simulink model "test_scenario"  (R2026a)
settings: Solver=FixedStepDiscrete  StopTime=inf  FixedStep=1/250
values from neighbouring files (symbols this model uses):
  amplitude_1 = 20e-6    (= 2e-05)    [STUBSCRIPT.m]    (also in main.m; main_calibrazione.m; profilazione.m; setup.m)
  amplitude_2 = 30e-6    (= 3e-05)    [STUBSCRIPT.m]    (also in main.m; main_calibrazione.m; profilazione.m; setup.m)
  amplitude_3 = 40e-6    (= 4e-05)    [STUBSCRIPT.m]    (also in main.m; main_calibrazione.m; profilazione.m; setup.m)
  amplitude_4 = 50e-6    (= 5e-05)    [STUBSCRIPT.m]    (also in main.m; main_calibrazione.m; profilazione.m; setup.m)
  unicorn_buff_size = 25    [STUBSCRIPT.m]    (also in main.m; main_calibrazione.m; profilazione.m; setup.m)
  unicorn_f = 250    [STUBSCRIPT.m]    (also in main.m; main_calibrazione.m; profilazione.m; setup.m)
undefined symbols (not defined in the file or in its folder): fdesignblkfcn, gcbh, UN
libraries: simulink x10, dspfdesign x8, dsparch4 x2, UnicornLib x1
settings Model: Creator=Utente  LastModifiedBy=Flexo Rodriguez

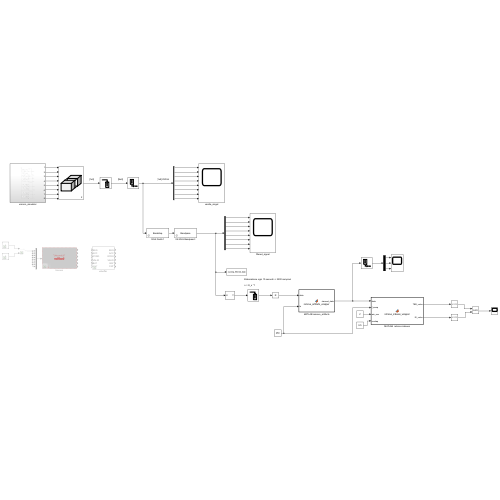
[thumbnail: Simulink's stored preview of the top-level diagram]
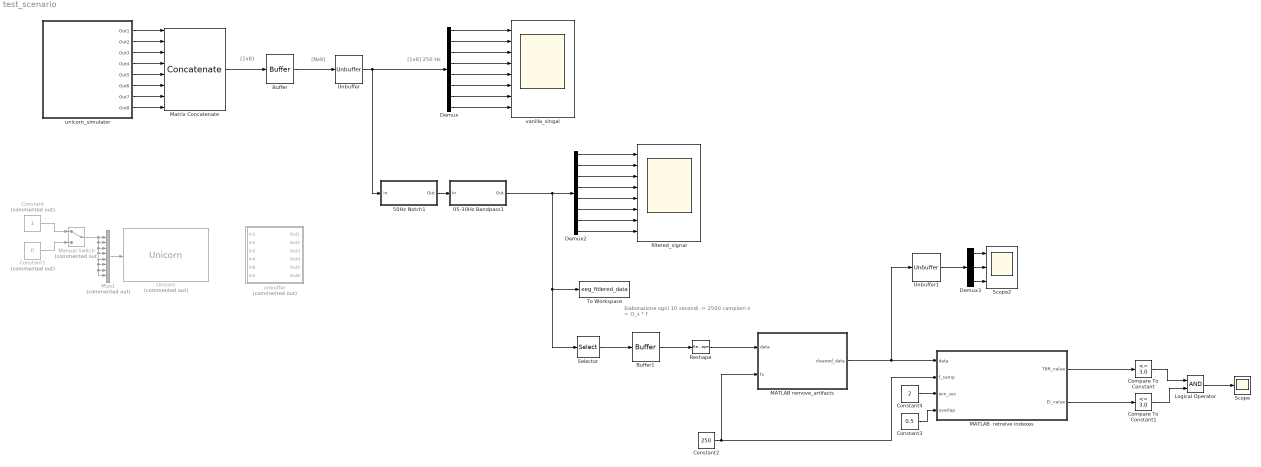
== system test_scenario ==
  note: Elaborazione ogni 10 secondi -> 2500 campioni
      |
      | n = O_s * f
  note: [1x8] 250 Hz
  note: [1x8]
  note: [Nx8]
  05-30Hz Bandpass1 : Subsystem  DialogController=fdesignblkfcn  InitFcn=fdesignblkfcn(gcbh, {'InitFcn'});  mask(Bandpass Filter){}
      mask help: Design a bandpass filter
      settings: CopyFcn=fdesignblkfcn(gcbh, {'CopyFcn'});
      mask Help: helpview(mapfilelocation('dsp'), 'dspbandpassfilter');
      mask Display: disp('Bandpass');
  50Hz Notch1 : Subsystem  DialogController=fdesignblkfcn  InitFcn=fdesignblkfcn(gcbh, {'InitFcn'});  mask(Bandstop Filter){}
      mask help: Design a bandstop filter
      settings: CopyFcn=fdesignblkfcn(gcbh, {'CopyFcn'});
      mask Help: helpview(mapfilelocation('dsp'), 'dspbandstopfilter');
      mask Display: disp('Bandstop');
  Buffer : Buffer  N=unicorn_buff_size  OutputFrames=off
  Buffer1 : Buffer  N=2500  OutputFrames=off
  Compare To Constant : simulink/Logic and Bit Operations/Compare To Constant  relop=<=  const=3.0  OutDataTypeStr=boolean
  Compare To Constant1 : simulink/Logic and Bit Operations/Compare To Constant  relop=<=  const=3.0  OutDataTypeStr=boolean
  Constant : Constant  Commented=on  OutDataTypeStr=boolean
  Constant1 : Constant  Commented=on  Value=0  OutDataTypeStr=boolean
  Constant2 : Constant  Value=250
  Constant3 : Constant  Value=0.5
  Constant4 : Constant  Value=2
  Demux : Demux  Outputs=8
  Demux2 : Demux  Outputs=8
  Demux3 : Demux  Outputs=3
  Logical Operator : Logic  AllPortsSameDT=off  OutDataTypeStr=boolean
  MATLAB  retreive indexes : MATLAB Function  TreatAsAtomicUnit=on
  MATLAB remove_artifacts : MATLAB Function  TreatAsAtomicUnit=on
  Manual Switch : ManualSwitch  Commented=on
  Matrix Concatenate : Concatenate  NumInputs=8  Mode=Multidimensional array  ConcatenateDimension=2
  Mux1 : Mux  Commented=on  Inputs=8
  Reshape : Reshape  OutputDimensionality=Customize  OutputDimensions=[2500,3]
  Scope : Scope
      settings: ActiveDisplayYMinimum=-1.7587335074953709  ActiveDisplayYMaximum=3.3735192626757464  DataLoggingVariableName=ScopeData2
  Scope2 : Scope  NumInputPorts=3
      settings: ActiveDisplayYMinimum=-2.8982593996217672  ActiveDisplayYMaximum=3.2740071294461224  DataLoggingVariableName=ScopeData4
  Selector : Selector  InputPortWidth=8  IndexOptions=Index vector (dialog)  Indices=[1 3 5]  OutputSizes=1
  To Workspace : ToWorkspace  VariableName=eeg_fitlered_data  SampleTime=-1
      settings: Save2DSignal=2-D array (concatenate along first dimension)
  Unbuffer : Unbuffer
  Unbuffer1 : Unbuffer
  Unicorn : UnicornLib/Unicorn  Commented=on  serial=UN-2023.04.40  old_serial=UN-2023.04.40  frame_length=1  input_source=Electrode
      settings: SourceProductName=Unicorn
  filtered_signal : Scope  NumInputPorts=8
      settings: ActiveDisplayYMinimum=-0.11132567955130231  ActiveDisplayYMaximum=0.12003241029464064  DataLoggingVariableName=ScopeData3
  "unbuffer " : Subsystem  Commented=on
      mask Display:
      | port_label('input',1,'EEG')
      | port_label('input',2,'ACC')
      | port_label('input',3,'GYRO')
      | port_label('input',4,'VALID')
      | port_label('input',5,'BAT')
      | port_label('input',6,'CNT')
      | port_label('output',1,'EEG')
      | port_label('output',2,'ACC')
      | port_label('output',3,'GYRO')
      | port_label('output',4,'VALID')
      | port_label('output',5,'BAT')
      | port_label('output',6,'CNT')
  unicorn_simulator : Subsystem
  vanilla_singal : Scope  NumInputPorts=8
      settings: ActiveDisplayString=4  ActiveDisplayYMinimum=-0.17938110629942738  ActiveDisplayYMaximum=0.15369010614959708
  wires:
  Constant/1 -> Manual Switch/1
  Mux1/1 -> Unicorn/1
  Manual Switch/1 -> Mux1/8, Mux1/7, Mux1/6, Mux1/5, Mux1/4, Mux1/3, Mux1/2, Mux1/1
  Constant1/1 -> Manual Switch/2
  unicorn_simulator/1(Out1) -> Matrix Concatenate/1
  unicorn_simulator/2(Out2) -> Matrix Concatenate/2
  unicorn_simulator/3(Out3) -> Matrix Concatenate/3
  unicorn_simulator/4(Out4) -> Matrix Concatenate/4
  unicorn_simulator/5(Out5) -> Matrix Concatenate/5
  unicorn_simulator/6(Out6) -> Matrix Concatenate/6
  unicorn_simulator/7(Out7) -> Matrix Concatenate/7
  unicorn_simulator/8(Out8) -> Matrix Concatenate/8
  Matrix Concatenate/1 -> Buffer/1
  Buffer/1 -> Unbuffer/1
  Unbuffer/1 -> Demux/1, 50Hz Notch1/1(In)
  Demux/1 -> vanilla_singal/1
  Demux/3 -> vanilla_singal/3
  Demux/2 -> vanilla_singal/2
  Demux/4 -> vanilla_singal/4
  Demux/5 -> vanilla_singal/5
  Demux/6 -> vanilla_singal/6
  Demux/7 -> vanilla_singal/7
  Demux/8 -> vanilla_singal/8
  50Hz Notch1/1(Out) -> 05-30Hz Bandpass1/1(In)
  05-30Hz Bandpass1/1(Out) -> Selector/1, To Workspace/1, Demux2/1
  Demux2/8 -> filtered_signal/8
  Demux2/3 -> filtered_signal/3
  Demux2/1 -> filtered_signal/1
  Demux2/7 -> filtered_signal/7
  Demux2/2 -> filtered_signal/2
  Demux2/4 -> filtered_signal/4
  Demux2/6 -> filtered_signal/6
  Demux2/5 -> filtered_signal/5
  Selector/1 -> Buffer1/1
  Constant2/1 -> MATLAB  retreive indexes/2(f_samp), MATLAB remove_artifacts/2(fs)
  MATLAB remove_artifacts/1(cleaned_data) -> Unbuffer1/1, MATLAB  retreive indexes/1(data)
  Constant4/1 -> MATLAB  retreive indexes/3(win_sec)
  Constant3/1 -> MATLAB  retreive indexes/4(overlap)
  Compare To Constant/1 -> Logical Operator/1
  Compare To Constant1/1 -> Logical Operator/2
  MATLAB  retreive indexes/1(TBR_value) -> Compare To Constant/1
  MATLAB  retreive indexes/2(EI_value) -> Compare To Constant1/1
  Logical Operator/1 -> Scope/1
  Buffer1/1 -> Reshape/1
  Reshape/1 -> MATLAB remove_artifacts/1(data)
  Demux3/1 -> Scope2/1
  Demux3/2 -> Scope2/2
  Demux3/3 -> Scope2/3
  Unbuffer1/1 -> Demux3/1

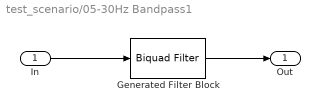
== system test_scenario/05-30Hz Bandpass1 ==
  In : Inport
  Generated Filter Block : dsparch4/Biquad Filter  Tag=BlockMethodSubSystem  FilterSource=Dialog parameters  CoeffSource=Specify via dialog  FilterObject=Hm_biquad  IIRFiltStruct=Direct form II  BiQuadCoeffs=[0.4322526152450743 0 -0.4322526152450743 1 -1.0011806751735479 0.3599418394747359;0.089147308745349971 0 -0.089147308745349971 1 -0.90316691443797437 0.21573805671244461;0.0088211325061849071 0 -0.0088211325061849071 1 -1.9935355151831708 0.99369356215971294;0.012337659349727709 0 -0.012337659349727709 1 -1.9822422643876501 0.98240374527709184;2 0 -2 1 -1.9751756853515128 0.97534142261558909;2 0 -2 1 -1.2458737431168365 0.70689135033598349]  ScaleValues=[0.35278894395693888;1;1;1;1;1;133.18750137787509]  IC=0  ICnum=0  ICden=0  a0Flag=Warning  optimizeScaleValues=on  ScaleValueMode=Specify via input port (g)  roundingMode=Floor  overflowMode=off  scaleValueFracLength=14  denProdOutputFracLength=30  denAccumFracLength=30  secondMemoryFracLength=15
  Out : Outport
  wires:
  In/1 -> Generated Filter Block/1
  Generated Filter Block/1 -> Out/1

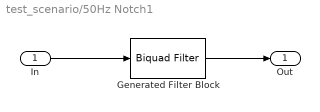
== system test_scenario/50Hz Notch1 ==
  In : Inport
  Generated Filter Block : dsparch4/Biquad Filter  Tag=BlockMethodSubSystem  FilterSource=Dialog parameters  CoeffSource=Specify via dialog  FilterObject=Hm_biquad  IIRFiltStruct=Direct form II  BiQuadCoeffs=[2 -1.2376311593598059 1.9999999999999996 1 -0.58917542534408363 0.90420359373902093]  ScaleValues=[0.091083863875771748;5.226511899890804]  IC=0  ICnum=0  ICden=0  a0Flag=Warning  optimizeScaleValues=on  ScaleValueMode=Specify via input port (g)  roundingMode=Floor  overflowMode=off  scaleValueFracLength=14  denProdOutputFracLength=30  denAccumFracLength=30  secondMemoryFracLength=15
  Out : Outport
  wires:
  Generated Filter Block/1 -> Out/1
  In/1 -> Generated Filter Block/1

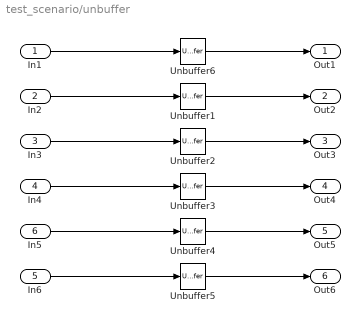
== system test_scenario/unbuffer  ==
  In1 : Inport
  In2 : Inport  Port=2
  In3 : Inport  Port=3
  In4 : Inport  Port=4
  In6 : Inport  Port=5
  In5 : Inport  Port=6
  Unbuffer{1..6} (6 alike) : Unbuffer
  Out1 : Outport
  Out2 : Outport  Port=2
  Out3 : Outport  Port=3
  Out4 : Outport  Port=4
  Out5 : Outport  Port=5
  Out6 : Outport  Port=6
  wires:
  In1/1 -> Unbuffer6/1
  In6/1 -> Unbuffer5/1
  In2/1 -> Unbuffer1/1
  In3/1 -> Unbuffer2/1
  In4/1 -> Unbuffer3/1
  In5/1 -> Unbuffer4/1
  Unbuffer4/1 -> Out5/1
  Unbuffer5/1 -> Out6/1
  Unbuffer3/1 -> Out4/1
  Unbuffer2/1 -> Out3/1
  Unbuffer1/1 -> Out2/1
  Unbuffer6/1 -> Out1/1

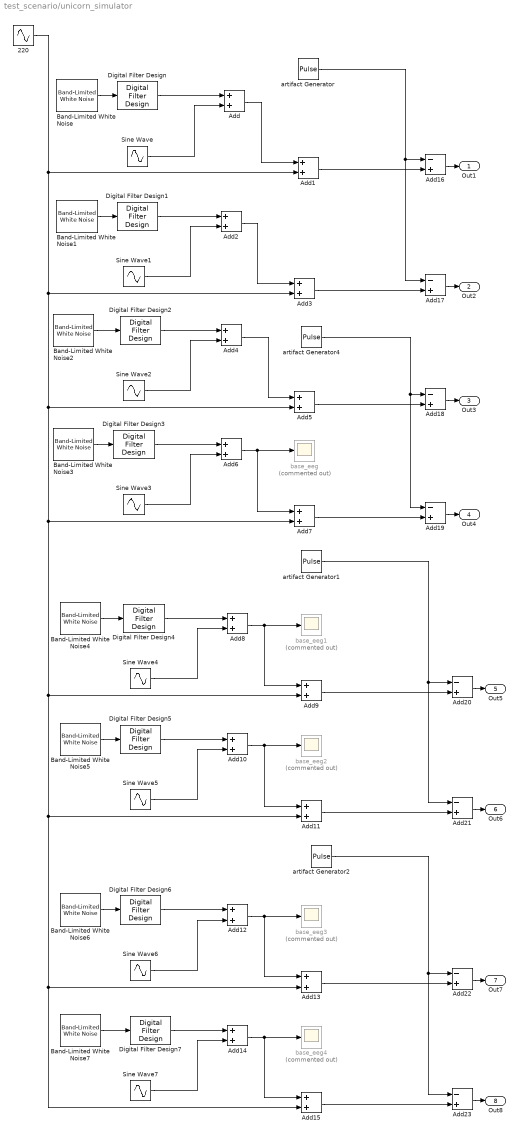
== system test_scenario/unicorn_simulator ==
  220 : Sin  SineType=Sample based  Amplitude=12e-6  Frequency=314.15  SampleTime=1/unicorn_f
  Add{,1..15} (16 alike) : Sum
  Add{16..23} (8 alike) : Sum  Inputs=-+
  Band-Limited White Noise : simulink/Sources/Band-Limited White Noise  Cov=[0.00001]  Ts=1/unicorn_f  seed=[23344]
  Band-Limited White Noise1 : simulink/Sources/Band-Limited White Noise  Cov=[0.00001]  Ts=1/unicorn_f  seed=[23344]
  Band-Limited White Noise2 : simulink/Sources/Band-Limited White Noise  Cov=[0.00001]  Ts=1/unicorn_f  seed=[23343]
  Band-Limited White Noise3 : simulink/Sources/Band-Limited White Noise  Cov=[0.00001]  Ts=1/unicorn_f  seed=[23343]
  Band-Limited White Noise4 : simulink/Sources/Band-Limited White Noise  Cov=[0.00001]  Ts=1/unicorn_f  seed=[23342]
  Band-Limited White Noise5 : simulink/Sources/Band-Limited White Noise  Cov=[0.00001]  Ts=1/unicorn_f  seed=[23342]
  Band-Limited White Noise6 : simulink/Sources/Band-Limited White Noise  Cov=[0.00001]  Ts=1/unicorn_f  seed=[23341]
  Band-Limited White Noise7 : simulink/Sources/Band-Limited White Noise  Cov=[0.00001]  Ts=1/unicorn_f  seed=[23341]
  Digital Filter Design{,1..7} (8 alike) : dspfdesign/Digital Filter Design  mwdsp_browser_bugfix_var=off
  Sine Wave : Sin  SineType=Sample based  Amplitude=amplitude_1  Frequency=62.83  SampleTime=1/unicorn_f
  Sine Wave1 : Sin  SineType=Sample based  Amplitude=amplitude_1  Frequency=62.83  SampleTime=1/unicorn_f
  Sine Wave2 : Sin  SineType=Sample based  Amplitude=amplitude_2  Frequency=62.83  SampleTime=1/unicorn_f
  Sine Wave3 : Sin  Amplitude=amplitude_2  Frequency=62.83  SampleTime=1/unicorn_f
  Sine Wave4 : Sin  SineType=Sample based  Amplitude=amplitude_3  Frequency=62.83  SampleTime=1/unicorn_f
  Sine Wave5 : Sin  SineType=Sample based  Amplitude=amplitude_3  Frequency=62.83  SampleTime=1/unicorn_f
  Sine Wave6 : Sin  SineType=Sample based  Amplitude=amplitude_4  Frequency=62.83  SampleTime=1/unicorn_f
  Sine Wave7 : Sin  SineType=Sample based  Amplitude=amplitude_4  Frequency=62.83  SampleTime=1/unicorn_f
  artifact Generator : DiscretePulseGenerator  Amplitude=1000*amplitude_1  Period=25000*(1/unicorn_f)  PulseWidth=30  SampleTime=1/unicorn_f
  artifact Generator1 : DiscretePulseGenerator  Amplitude=1000*amplitude_3  Period=25000*(1/unicorn_f)  PulseWidth=30  SampleTime=1/unicorn_f
  artifact Generator2 : DiscretePulseGenerator  Amplitude=1000*amplitude_4  Period=25000*(1/unicorn_f)  PulseWidth=30  SampleTime=1/unicorn_f
  artifact Generator4 : DiscretePulseGenerator  Amplitude=1000*amplitude_2  Period=25000*(1/unicorn_f)  PulseWidth=30  SampleTime=1/unicorn_f
  base_eeg{,1..4} (5 alike) : Scope  Commented=on
      base_eeg settings: ActiveDisplayYMinimum=-0.035555269827580581  ActiveDisplayYMaximum=0.026072132085607332
      base_eeg1 settings: ActiveDisplayYMinimum=-0.035555269827580581  ActiveDisplayYMaximum=0.026072132085607332  DataLoggingVariableName=ScopeData5
      base_eeg2 settings: ActiveDisplayYMinimum=-0.035555269827580581  ActiveDisplayYMaximum=0.026072132085607332  DataLoggingVariableName=ScopeData7
      base_eeg3 settings: ActiveDisplayYMinimum=-0.035555269827580581  ActiveDisplayYMaximum=0.026072132085607332  DataLoggingVariableName=ScopeData9
      base_eeg4 settings: ActiveDisplayYMinimum=-0.035555269827580581  ActiveDisplayYMaximum=0.026072132085607332  DataLoggingVariableName=ScopeData11
  Out1 : Outport
  Out2 : Outport  Port=2
  Out3 : Outport  Port=3
  Out4 : Outport  Port=4
  Out5 : Outport  Port=5
  Out6 : Outport  Port=6
  Out7 : Outport  Port=7
  Out8 : Outport  Port=8
  wires:
  Add1/1 -> Add16/2
  Digital Filter Design2/1 -> Add4/1
  Band-Limited White Noise7/1 -> Digital Filter Design7/1
  Sine Wave/1 -> Add/2
  Digital Filter Design4/1 -> Add8/1
  Add/1 -> Add1/1
  Digital Filter Design1/1 -> Add2/1
  220/1 -> Add15/2, Add13/2, Add11/2, Add9/2, Add7/2, Add5/2, Add3/2, Add1/2
  Digital Filter Design6/1 -> Add12/1
  Band-Limited White Noise6/1 -> Digital Filter Design6/1
  Add5/1 -> Add18/2
  Add18/1 -> Out3/1
  Add20/1 -> Out5/1
  artifact Generator4/1 -> Add19/1, Add18/1
  Sine Wave1/1 -> Add2/2
  Sine Wave3/1 -> Add6/2
  Add9/1 -> Add20/2
  Add16/1 -> Out1/1
  Add7/1 -> Add19/2
  Add13/1 -> Add22/2
  Add8/1 -> Add9/1, base_eeg1/1
  Band-Limited White Noise2/1 -> Digital Filter Design2/1
  Add15/1 -> Add23/2
  artifact Generator2/1 -> Add22/1, Add23/1
  Add2/1 -> Add3/1
  Add6/1 -> Add7/1, base_eeg/1
  Add4/1 -> Add5/1
  Band-Limited White Noise1/1 -> Digital Filter Design1/1
  Band-Limited White Noise5/1 -> Digital Filter Design5/1
  Band-Limited White Noise4/1 -> Digital Filter Design4/1
  Digital Filter Design7/1 -> Add14/1
  artifact Generator1/1 -> Add21/1, Add20/1
  Add12/1 -> Add13/1, base_eeg3/1
  artifact Generator/1 -> Add16/1, Add17/1
  Add3/1 -> Add17/2
  Add14/1 -> Add15/1, base_eeg4/1
  Add11/1 -> Add21/2
  Digital Filter Design5/1 -> Add10/1
  Sine Wave2/1 -> Add4/2
  Sine Wave7/1 -> Add14/2
  Sine Wave4/1 -> Add8/2
  Sine Wave5/1 -> Add10/2
  Sine Wave6/1 -> Add12/2
  Add10/1 -> Add11/1, base_eeg2/1
  Add22/1 -> Out7/1
  Add19/1 -> Out4/1
  Add23/1 -> Out8/1
  Add17/1 -> Out2/1
  Add21/1 -> Out6/1
  Band-Limited White Noise/1 -> Digital Filter Design/1
  Digital Filter Design/1 -> Add/1
  Band-Limited White Noise3/1 -> Digital Filter Design3/1
  Digital Filter Design3/1 -> Add6/1

== matlab function test_scenario/MATLAB  retreive indexes ==
  data: data input; TBR_value output; f_samp input; win_sec input; overlap input; EI_value output
function [TBR_value, EI_value] = retrieve_indexes_wrapper(data,f_samp,win_sec, overlap)
    coder.extrinsic('utils.retrieve_indexes_fly');
    TBR_value = double(0);
    EI_value = double(0);
    [TBR_value, EI_value] = utils.retrieve_indexes_fly(data, f_samp, win_sec, overlap);

== matlab function test_scenario/MATLAB remove_artifacts ==
  data: data input; cleaned_data output; fs input
function cleaned_data = remove_artifacts_wrapper(data, fs)
    coder.extrinsic('utils.remove_artifacts_eeg_fly');

    cleaned_data = zeros(2500, 3); 
    cleaned_data = utils.remove_artifacts_eeg_fly(data, fs);
end
